simulink model "scale_model_model_control"  (R2024b)
settings: Solver=VariableStepAuto  StartTime=0.0  StopTime=100  MaxStep=0.02  RelTol=1e-3
values from neighbouring files (symbols this model uses):
  A_adrcl = [zeros(N, 1)  eye(N, N) ... (first row only)    [init_scale_blade_suspended_control.m]
  A_ESO_d = [1-l1_ESO_d, delta_t-l1_ESO_d*delta_t, 1/2 * delta_t^2 - 1/2 * l1_ESO_d*delta_t^2 ... (first row only)    [init_scale_blade_suspended_control.m]
  A_MESO_d = A_o_d - l_MESO_d*C_o_d*A_o_d    [init_scale_blade_suspended_control.m]
  b0 = 1.025    [init_scale_blade_suspended_control.m]
  b_adrcl = [zeros(N-1, 1) ... (first row only)    [init_scale_blade_suspended_control.m]
  b_ESO_d = [1/2*b0*delta_t^2 - l1_ESO_d*b0*delta_t^2 ... (first row only)    [init_scale_blade_suspended_control.m]
  B_MESO_d = B_o_d - l_MESO_d*C_o_d*B_o_d    [init_scale_blade_suspended_control.m]
  c_t = [1, zeros(1, N)]    [init_scale_blade_suspended_control.m]
  delta_t = 0.01    [init_scale_blade_suspended_control.m]
  DLADRC_max_effort = 30    [init_scale_blade_suspended_control.m]
  DLQRMADRC_max_effort = 30    [init_scale_blade_suspended_control.m]
  eta_s_init_n = [p_s_init_n;Theta_s_init_n]    [init_scale_blade_suspended_control.m]
  g = 9.81    [init_scale_blade_suspended_control.m]
  inv_M_s = inv(M_s)    [init_scale_blade_suspended_control.m]
  k = ones(N,1)    [init_scale_blade_suspended_control.m]
  k1_c_d = (1 - z_cl)^2/delta_t^2    [init_scale_blade_suspended_control.m]
  k_c_T_dlqr = dlqr(A_m_dlqr,b_m_dlqr,Q,R)    [init_scale_blade_suspended_control.m]
  k_d_T_lqr = (e_m*c_T_d_m_lqr) \ b_m_lqr    [init_scale_blade_suspended_control.m]
  k_s_lqr = -inv(c_T_m_lqr*inv(A_m_lqr-b_m_lqr*k_c_T_lqr)*b_m_lqr)    [init_scale_blade_suspended_control.m]
  k_T_d = [k1_c_d, k2_c_d]    [init_scale_blade_suspended_control.m]
  k_w1_s = gamma * EA/lw1_s_init    (= 19634.9540849)    [init_scale_blade_suspended_control.m]
  k_w2_s = k_w1_s    (= 19634.9540849)    [init_scale_blade_suspended_control.m]
  L = 0.8    [init_scale_blade_suspended_control.m]
  l = ones(N+1, 1)    [init_scale_blade_suspended_control.m]
  l_ESO_d = [l1_ESO_d, l2_ESO_d, l3_ESO_d]'    [init_scale_blade_suspended_control.m]
  l_MESO_d = acker(A_o_d',C_o_d',[z_MESO,z_MESO,z_MESO])'    [init_scale_blade_suspended_control.m]
  lw1_s_init = tot_liftWire-0.14    (= 0.56)    [init_scale_blade_suspended_control.m]
  lw2_s = norm(p_h_s_init- posSling_s_n(:,1))-elong_lw2_s    [init_scale_blade_suspended_control.m]
  m_h_s = 0.01    [init_scale_blade_suspended_control.m]
  meanWSP = 1    [init_scale_blade_suspended_control.m]
  N = 2    [init_scale_blade_suspended_control.m]
  nu_s_init_b = zeros(6,1)    [init_scale_blade_suspended_control.m]
  p_h_dot_s_init = [0;0;0]    [init_scale_blade_suspended_control.m]
  p_h_s_init = posCraneTip_s + [0;0;lw1_s_init + elong_mainlw_s]    [init_scale_blade_suspended_control.m]
  posCOG_s = [0;0;0]    [init_scale_blade_suspended_control.m]
  posCraneTip_s = [0;0;-1.2]    [init_scale_blade_suspended_control.m]
  posSling_s_b = [posCOG_s + [slings_p1_new(1); -0.05; slings_p1_new(2)],                posCOG_s + [slings_p1_new(1); 0.05; slings_p1_new(2)],               posCOG_s + [slings_p2_new(1); -0.05; slings_p2_new(2)],               posCOG_s + [slings_p2_new(1); 0.05; slings_p2_new(2)]]    [init_scale_blade_suspended_control.m]
  posThruster_s_b = [posCOG_s + [0.03; 0.21; -0.05],                posCOG_s + [0.03; -0.21; -0.05],               posCOG_s + [0; 0.1825; -0.05],               posCOG_s + [0; -0.1825; -0.05]]    [init_scale_blade_suspended_control.m]
  totalMass_s = 0.391    [init_scale_blade_suspended_control.m]
  W = 0.05    [init_scale_blade_suspended_control.m]
undefined symbols (not defined in the file or in its folder): A_o_dlqr, b_o_dlqr, c_o_T_dlqr, k_o_lqr, linsys_v2, sigbuilder_block
libraries: MarIn_blade x104, simulink_extras x28, slpidlib x5, simulink x4
(part 2 of 3)

== system scale_model_model_control/Discrete LADRC ==
  note: Discrete ESO
  ref : Inport
  y : Inport  Port=2
  Gain : Gain  Gain=l_ESO_d
  Gain1 : Gain  Gain=b_ESO_d
  Gain2 : Gain  Gain=A_ESO_d  Multiplication=Matrix(K*u)
  Gain3 : Gain  Gain=k1_c_d
  Gain4 : Gain  Gain=1/b0
  Gain5 : Gain  Gain=[k_T_d 1]  Multiplication=Matrix(K*u)
  Limiter : Saturate  UpperLimit=DLADRC_max_effort  LowerLimit=-DLADRC_max_effort
  Sum : Sum  Inputs=|+-
  Sum8 : Sum  Inputs=|++
  Sum9 : Sum  Inputs=+|+
  Unit Delay : UnitDelay  SampleTime=delta_t  HasFrameUpgradeWarning=on
  u : Outport
  wires:
  Gain1/1 -> Sum8/1
  Unit Delay/1 -> Sum9/1
  Sum8/1 -> Unit Delay/1
  Sum9/1 -> Gain5/1, Gain2/1  "x_hat"
  Gain/1 -> Sum9/2
  Gain2/1 -> Sum8/2
  Gain4/1 -> Limiter/1  "u"
  ref/1 -> Gain3/1
  Gain3/1 -> Sum/1
  Sum/1 -> Gain4/1
  Limiter/1 -> Gain1/1, u/1  "u_lim"
  y/1 -> Gain/1
  Gain5/1 -> Sum/2

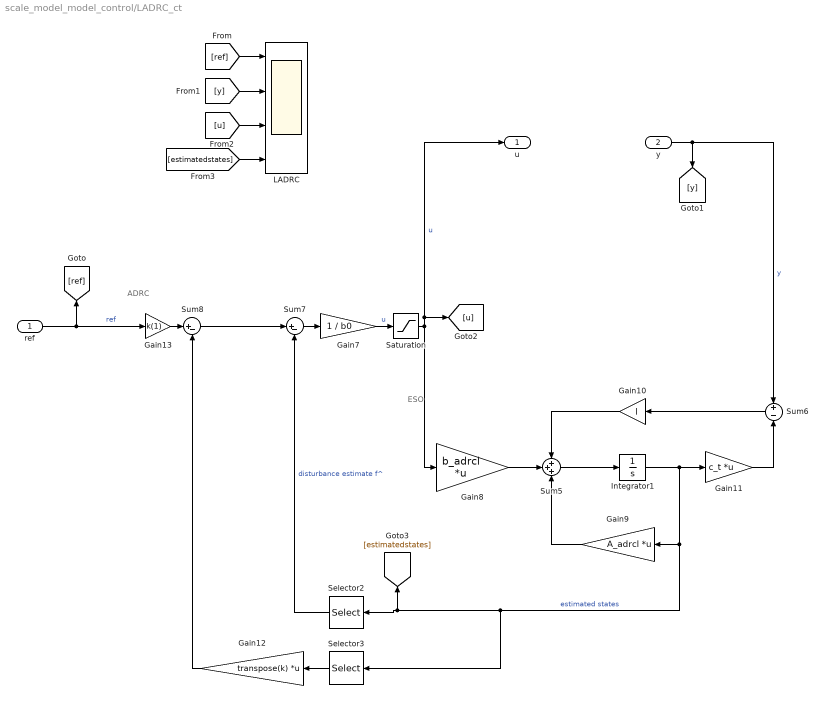
== system scale_model_model_control/LADRC_ct ==
  note: ESO
  note: ADRC
  ref : Inport
  y : Inport  Port=2
  Gain10 : Gain  Gain=l
  Gain11 : Gain  Gain=c_t  Multiplication=Matrix(K*u)
  Gain12 : Gain  Gain=transpose(k)  Multiplication=Matrix(K*u)
  Gain13 : Gain  Gain=k(1)
  Gain7 : Gain  Gain=1 / b0
  Gain8 : Gain  Gain=b_adrcl  Multiplication=Matrix(K*u)
  Gain9 : Gain  Gain=A_adrcl  Multiplication=Matrix(K*u)
  Integrator1 : Integrator
  LADRC : Scope  NumInputPorts=4
  Saturation : Saturate
  Selector2 : Selector  InputPortWidth=N+1  IndexOptions=Index vector (dialog)  Indices=[N+1]  OutputSizes=1
  Selector3 : Selector  InputPortWidth=N+1  IndexOptions=Index vector (dialog)  Indices=[1:N]  OutputSizes=1
  Sum5 : Sum  Inputs=+++
  Sum6 : Sum  Inputs=+|-
  Sum7 : Sum  Inputs=|+-
  Sum8 : Sum  Inputs=|+-
  u : Outport
  wires:
  Gain8/1 -> Sum5/2
  Saturation/1 -> u/1, [u], Gain8/1  "u"
  Integrator1/1 -> Gain11/1, Selector3/1, [estimatedstates], Selector2/1, Gain9/1  "estimated states"
  Gain11/1 -> Sum6/2
  Sum6/1 -> Gain10/1
  Selector2/1 -> Sum7/2  "disturbance estimate f^"
  Sum7/1 -> Gain7/1
  Gain12/1 -> Sum8/2
  Gain10/1 -> Sum5/1
  Gain9/1 -> Sum5/3
  Gain13/1 -> Sum8/1
  Sum5/1 -> Integrator1/1
  Selector3/1 -> Gain12/1
  Sum8/1 -> Sum7/1
  ref/1 -> [ref], Gain13/1  "ref"
  y/1 -> Sum6/1, [y]  "y"
  [ref] -> LADRC/1
  [y] -> LADRC/2
  [u] -> LADRC/3
  [estimatedstates] -> LADRC/4
  Gain7/1 -> Saturation/1  "u"

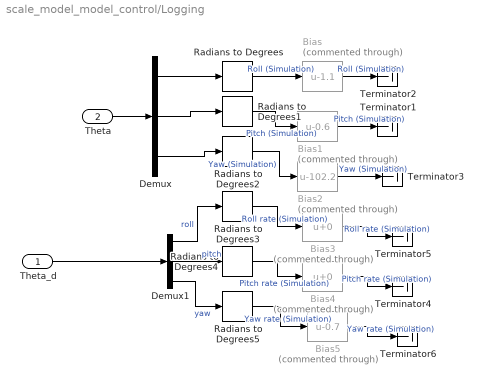
== system scale_model_model_control/Logging ==
  Theta_d : Inport
  Theta : Inport  Port=2
  Bias : Bias  Commented=through  Bias=-1.1  SaturateOnIntegerOverflow=off
  Bias1 : Bias  Commented=through  Bias=-0.6  SaturateOnIntegerOverflow=off
  Bias2 : Bias  Commented=through  Bias=-102.2  SaturateOnIntegerOverflow=off
  Bias3 : Bias  Commented=through  SaturateOnIntegerOverflow=off
  Bias4 : Bias  Commented=through  SaturateOnIntegerOverflow=off
  Bias5 : Bias  Commented=through  Bias=-0.7  SaturateOnIntegerOverflow=off
  Demux : Demux  Outputs=3
  Demux1 : Demux  Outputs=3
  Radians to Degrees{,1..5} (6 alike) : simulink_extras/Transformations/Radians to Degrees
  Terminator{1..6} (6 alike) : Terminator
  wires:
  Bias5/1 -> Terminator6/1  "Yaw rate (Simulation)"
  Bias2/1 -> Terminator3/1  "Yaw (Simulation)"
  Radians to Degrees3/1 -> Bias3/1  "Roll rate (Simulation)"
  Radians to Degrees5/1 -> Bias5/1  "Yaw rate (Simulation)"
  Bias/1 -> Terminator2/1  "Roll (Simulation)"
  Radians to Degrees/1 -> Bias/1  "Roll (Simulation)"
  Bias3/1 -> Terminator5/1  "Roll rate (Simulation)"
  Radians to Degrees4/1 -> Bias4/1  "Pitch rate (Simulation)"
  Demux1/3 -> Radians to Degrees5/1  "yaw"
  Demux1/1 -> Radians to Degrees3/1  "roll"
  Radians to Degrees2/1 -> Bias2/1  "Yaw (Simulation)"
  Bias4/1 -> Terminator4/1  "Pitch rate (Simulation)"
  Bias1/1 -> Terminator1/1  "Pitch (Simulation)"
  Radians to Degrees1/1 -> Bias1/1  "Pitch (Simulation)"
  Demux1/2 -> Radians to Degrees4/1  "pitch"
  Theta_d/1 -> Demux1/1
  Theta/1 -> Demux/1
  Demux/1 -> Radians to Degrees/1
  Demux/2 -> Radians to Degrees1/1
  Demux/3 -> Radians to Degrees2/1

== system scale_model_model_control/Logging1 ==
  Theta_d : Inport
  Theta : Inport  Port=2
  Bias : Bias  Commented=through  Bias=-1.1  SaturateOnIntegerOverflow=off
  Bias1 : Bias  Commented=through  Bias=-0.6  SaturateOnIntegerOverflow=off
  Bias2 : Bias  Commented=through  Bias=-102.2  SaturateOnIntegerOverflow=off
  Bias3 : Bias  Commented=through  SaturateOnIntegerOverflow=off
  Bias4 : Bias  Commented=through  SaturateOnIntegerOverflow=off
  Bias5 : Bias  Commented=through  Bias=-0.7  SaturateOnIntegerOverflow=off
  Demux : Demux  Outputs=3
  Demux1 : Demux  Outputs=3
  Radians to Degrees{,1..5} (6 alike) : simulink_extras/Transformations/Radians to Degrees
  Terminator{1..6} (6 alike) : Terminator
  wires:
  Bias5/1 -> Terminator6/1  "Yaw rate (Simulation)"
  Bias2/1 -> Terminator3/1  "Yaw (Simulation)"
  Radians to Degrees3/1 -> Bias3/1  "Roll rate (Simulation)"
  Radians to Degrees5/1 -> Bias5/1  "Yaw rate (Simulation)"
  Bias/1 -> Terminator2/1  "Roll (Simulation)"
  Radians to Degrees/1 -> Bias/1  "Roll (Simulation)"
  Bias3/1 -> Terminator5/1  "Roll rate (Simulation)"
  Radians to Degrees4/1 -> Bias4/1  "Pitch rate (Simulation)"
  Demux1/3 -> Radians to Degrees5/1  "yaw"
  Demux1/1 -> Radians to Degrees3/1  "roll"
  Radians to Degrees2/1 -> Bias2/1  "Yaw (Simulation)"
  Bias4/1 -> Terminator4/1  "Pitch rate (Simulation)"
  Bias1/1 -> Terminator1/1  "Pitch (Simulation)"
  Radians to Degrees1/1 -> Bias1/1  "Pitch (Simulation)"
  Demux1/2 -> Radians to Degrees4/1  "pitch"
  Theta_d/1 -> Demux1/1
  Theta/1 -> Demux/1
  Demux/1 -> Radians to Degrees/1
  Demux/2 -> Radians to Degrees1/1
  Demux/3 -> Radians to Degrees2/1

== system scale_model_model_control/Logging2 ==
  Theta_d : Inport
  Theta : Inport  Port=2
  Bias : Bias  Commented=through  Bias=-1.1  SaturateOnIntegerOverflow=off
  Bias1 : Bias  Commented=through  Bias=-0.6  SaturateOnIntegerOverflow=off
  Bias2 : Bias  Commented=through  Bias=-102.2  SaturateOnIntegerOverflow=off
  Bias3 : Bias  Commented=through  SaturateOnIntegerOverflow=off
  Bias4 : Bias  Commented=through  SaturateOnIntegerOverflow=off
  Bias5 : Bias  Commented=through  Bias=-0.7  SaturateOnIntegerOverflow=off
  Demux : Demux  Outputs=3
  Demux1 : Demux  Outputs=3
  Radians to Degrees{,1..5} (6 alike) : simulink_extras/Transformations/Radians to Degrees
  Terminator{1..6} (6 alike) : Terminator
  wires:
  Bias5/1 -> Terminator6/1  "Yaw rate (Simulation)"
  Bias2/1 -> Terminator3/1  "Yaw (Simulation)"
  Radians to Degrees3/1 -> Bias3/1  "Roll rate (Simulation)"
  Radians to Degrees5/1 -> Bias5/1  "Yaw rate (Simulation)"
  Bias/1 -> Terminator2/1  "Roll (Simulation)"
  Radians to Degrees/1 -> Bias/1  "Roll (Simulation)"
  Bias3/1 -> Terminator5/1  "Roll rate (Simulation)"
  Radians to Degrees4/1 -> Bias4/1  "Pitch rate (Simulation)"
  Demux1/3 -> Radians to Degrees5/1  "yaw"
  Demux1/1 -> Radians to Degrees3/1  "roll"
  Radians to Degrees2/1 -> Bias2/1  "Yaw (Simulation)"
  Bias4/1 -> Terminator4/1  "Pitch rate (Simulation)"
  Bias1/1 -> Terminator1/1  "Pitch (Simulation)"
  Radians to Degrees1/1 -> Bias1/1  "Pitch (Simulation)"
  Demux1/2 -> Radians to Degrees4/1  "pitch"
  Theta_d/1 -> Demux1/1
  Theta/1 -> Demux/1
  Demux/1 -> Radians to Degrees/1
  Demux/2 -> Radians to Degrees1/1
  Demux/3 -> Radians to Degrees2/1

== system scale_model_model_control/Logging3 ==
  Theta_d : Inport
  Theta : Inport  Port=2
  Bias : Bias  Commented=through  Bias=-1.1  SaturateOnIntegerOverflow=off
  Bias1 : Bias  Commented=through  Bias=-0.6  SaturateOnIntegerOverflow=off
  Bias2 : Bias  Commented=through  Bias=-102.2  SaturateOnIntegerOverflow=off
  Bias3 : Bias  Commented=through  SaturateOnIntegerOverflow=off
  Bias4 : Bias  Commented=through  SaturateOnIntegerOverflow=off
  Bias5 : Bias  Commented=through  Bias=-0.7  SaturateOnIntegerOverflow=off
  Demux : Demux  Outputs=3
  Demux1 : Demux  Outputs=3
  Radians to Degrees{,1..5} (6 alike) : simulink_extras/Transformations/Radians to Degrees
  Terminator{1..6} (6 alike) : Terminator
  wires:
  Bias5/1 -> Terminator6/1  "Yaw rate (Simulation)"
  Bias2/1 -> Terminator3/1  "Yaw (Simulation)"
  Radians to Degrees3/1 -> Bias3/1  "Roll rate (Simulation)"
  Radians to Degrees5/1 -> Bias5/1  "Yaw rate (Simulation)"
  Bias/1 -> Terminator2/1  "Roll (Simulation)"
  Radians to Degrees/1 -> Bias/1  "Roll (Simulation)"
  Bias3/1 -> Terminator5/1  "Roll rate (Simulation)"
  Radians to Degrees4/1 -> Bias4/1  "Pitch rate (Simulation)"
  Demux1/3 -> Radians to Degrees5/1  "yaw"
  Demux1/1 -> Radians to Degrees3/1  "roll"
  Radians to Degrees2/1 -> Bias2/1  "Yaw (Simulation)"
  Bias4/1 -> Terminator4/1  "Pitch rate (Simulation)"
  Bias1/1 -> Terminator1/1  "Pitch (Simulation)"
  Radians to Degrees1/1 -> Bias1/1  "Pitch (Simulation)"
  Demux1/2 -> Radians to Degrees4/1  "pitch"
  Theta_d/1 -> Demux1/1
  Theta/1 -> Demux/1
  Demux/1 -> Radians to Degrees/1
  Demux/2 -> Radians to Degrees1/1
  Demux/3 -> Radians to Degrees2/1

== system scale_model_model_control/Thrusters ==
  M_Tx : Inport
  M_Tz : Inport  Port=2
  Abs : Abs  SaturateOnIntegerOverflow=off
  Abs1 : Abs  SaturateOnIntegerOverflow=off
  Constant : Constant  Value=0
  Constant1 : Constant  Value=posThruster_s_b(2,2)
  Divide : Product  Inputs=*/
  Divide1 : Product  Inputs=*/
  Max F_t ~0.3N : Saturate  UpperLimit=0.076  LowerLimit=-0.076  LinearizeAsGain=off
  Mux : Mux
  Mux{1..4} (4 alike) : Mux  Inputs=3
  Saturation : Saturate  UpperLimit=0  LowerLimit=-inf
  Saturation1 : Saturate  UpperLimit=inf  LowerLimit=0
  Saturation2 : Saturate  UpperLimit=0  LowerLimit=-inf
  Saturation3 : Saturate  UpperLimit=inf  LowerLimit=0
  "F_thrusters {b}" : Outport
  wires:
  Mux1/1 -> Mux/1  "thruster1 (yaw)"
  Mux2/1 -> Mux/2  "thruster2 (yaw)"
  Mux3/1 -> Mux/3  "thruster3 (roll)"
  Mux4/1 -> Mux/4  "thruster4 (roll)"
  Constant/1 -> Mux1/3, Mux3/1, Mux4/2, Mux4/1, Mux3/2, Mux2/3, Mux2/2, Mux1/2
  M_Tx/1 -> Divide/1
  Constant1/1 -> Divide1/2, Divide/2
  M_Tz/1 -> Divide1/1
  Divide1/1 -> Saturation/1, Saturation1/1
  Saturation1/1 -> Mux1/1
  Saturation/1 -> Abs1/1
  Divide/1 -> Saturation2/1, Saturation3/1
  Saturation3/1 -> Mux4/3
  Saturation2/1 -> Abs/1
  Abs/1 -> Mux3/3
  Abs1/1 -> Mux2/1
  Mux/1 -> Max F_t ~0.3N/1
  Max F_t ~0.3N/1 -> "F_thrusters {b}"/1  "F_T"

== system scale_model_model_control/Thrusters1 ==
  M_Tx : Inport
  M_Tz : Inport  Port=2
  Abs : Abs  SaturateOnIntegerOverflow=off
  Abs1 : Abs  SaturateOnIntegerOverflow=off
  Constant : Constant  Value=0
  Constant1 : Constant  Value=posThruster_s_b(2,2)
  Divide : Product  Inputs=*/
  Divide1 : Product  Inputs=*/
  Max F_t ~0.3N : Saturate  UpperLimit=0.076  LowerLimit=-0.076  LinearizeAsGain=off
  Mux : Mux
  Mux{1..4} (4 alike) : Mux  Inputs=3
  Saturation : Saturate  UpperLimit=0  LowerLimit=-inf
  Saturation1 : Saturate  UpperLimit=inf  LowerLimit=0
  Saturation2 : Saturate  UpperLimit=0  LowerLimit=-inf
  Saturation3 : Saturate  UpperLimit=inf  LowerLimit=0
  "F_thrusters {b}" : Outport
  wires:
  Mux1/1 -> Mux/1  "thruster1 (yaw)"
  Mux2/1 -> Mux/2  "thruster2 (yaw)"
  Mux3/1 -> Mux/3  "thruster3 (roll)"
  Mux4/1 -> Mux/4  "thruster4 (roll)"
  Constant/1 -> Mux1/3, Mux3/1, Mux4/2, Mux4/1, Mux3/2, Mux2/3, Mux2/2, Mux1/2
  M_Tx/1 -> Divide/1
  Constant1/1 -> Divide1/2, Divide/2
  M_Tz/1 -> Divide1/1
  Divide1/1 -> Saturation/1, Saturation1/1
  Saturation1/1 -> Mux1/1
  Saturation/1 -> Abs1/1
  Divide/1 -> Saturation2/1, Saturation3/1
  Saturation3/1 -> Mux4/3
  Saturation2/1 -> Abs/1
  Abs/1 -> Mux3/3
  Abs1/1 -> Mux2/1
  Mux/1 -> Max F_t ~0.3N/1
  Max F_t ~0.3N/1 -> "F_thrusters {b}"/1  "F_T"

== system scale_model_model_control/Thrusters2 ==
  M_Tx : Inport
  M_Tz : Inport  Port=2
  Abs : Abs  SaturateOnIntegerOverflow=off
  Abs1 : Abs  SaturateOnIntegerOverflow=off
  Constant : Constant  Value=0
  Constant1 : Constant  Value=posThruster_s_b(2,2)
  Divide : Product  Inputs=*/
  Divide1 : Product  Inputs=*/
  Max F_t ~0.3N : Saturate  UpperLimit=0.076  LowerLimit=-0.076  LinearizeAsGain=off
  Mux : Mux
  Mux{1..4} (4 alike) : Mux  Inputs=3
  Saturation : Saturate  UpperLimit=0  LowerLimit=-inf
  Saturation1 : Saturate  UpperLimit=inf  LowerLimit=0
  Saturation2 : Saturate  UpperLimit=0  LowerLimit=-inf
  Saturation3 : Saturate  UpperLimit=inf  LowerLimit=0
  "F_thrusters {b}" : Outport
  wires:
  Mux1/1 -> Mux/1  "thruster1 (yaw)"
  Mux2/1 -> Mux/2  "thruster2 (yaw)"
  Mux3/1 -> Mux/3  "thruster3 (roll)"
  Mux4/1 -> Mux/4  "thruster4 (roll)"
  Constant/1 -> Mux1/3, Mux3/1, Mux4/2, Mux4/1, Mux3/2, Mux2/3, Mux2/2, Mux1/2
  M_Tx/1 -> Divide/1
  Constant1/1 -> Divide1/2, Divide/2
  M_Tz/1 -> Divide1/1
  Divide1/1 -> Saturation/1, Saturation1/1
  Saturation1/1 -> Mux1/1
  Saturation/1 -> Abs1/1
  Divide/1 -> Saturation2/1, Saturation3/1
  Saturation3/1 -> Mux4/3
  Saturation2/1 -> Abs/1
  Abs/1 -> Mux3/3
  Abs1/1 -> Mux2/1
  Mux/1 -> Max F_t ~0.3N/1
  Max F_t ~0.3N/1 -> "F_thrusters {b}"/1  "F_T"

== system scale_model_model_control/Thrusters3 ==
  M_Tx : Inport
  M_Tz : Inport  Port=2
  Abs : Abs  SaturateOnIntegerOverflow=off
  Abs1 : Abs  SaturateOnIntegerOverflow=off
  Constant : Constant  Value=0
  Constant1 : Constant  Value=posThruster_s_b(2,2)
  Divide : Product  Inputs=*/
  Divide1 : Product  Inputs=*/
  Max F_t ~0.3N : Saturate  UpperLimit=0.076  LowerLimit=-0.076  LinearizeAsGain=off
  Mux : Mux
  Mux{1..4} (4 alike) : Mux  Inputs=3
  Saturation : Saturate  UpperLimit=0  LowerLimit=-inf
  Saturation1 : Saturate  UpperLimit=inf  LowerLimit=0
  Saturation2 : Saturate  UpperLimit=0  LowerLimit=-inf
  Saturation3 : Saturate  UpperLimit=inf  LowerLimit=0
  "F_thrusters {b}" : Outport
  wires:
  Mux1/1 -> Mux/1  "thruster1 (yaw)"
  Mux2/1 -> Mux/2  "thruster2 (yaw)"
  Mux3/1 -> Mux/3  "thruster3 (roll)"
  Mux4/1 -> Mux/4  "thruster4 (roll)"
  Constant/1 -> Mux1/3, Mux3/1, Mux4/2, Mux4/1, Mux3/2, Mux2/3, Mux2/2, Mux1/2
  M_Tx/1 -> Divide/1
  Constant1/1 -> Divide1/2, Divide/2
  M_Tz/1 -> Divide1/1
  Divide1/1 -> Saturation/1, Saturation1/1
  Saturation1/1 -> Mux1/1
  Saturation/1 -> Abs1/1
  Divide/1 -> Saturation2/1, Saturation3/1
  Saturation3/1 -> Mux4/3
  Saturation2/1 -> Abs/1
  Abs/1 -> Mux3/3
  Abs1/1 -> Mux2/1
  Mux/1 -> Max F_t ~0.3N/1
  Max F_t ~0.3N/1 -> "F_thrusters {b}"/1  "F_T"

== system scale_model_model_control/Blade+Yoke/Signal Builder2 ==
  Demux : Demux  Tag=STV Demux  Outputs=1
      settings: DisplayOption=none
  FromWs : FromWorkspace  Tag=STV FromWs  VariableName=tuvar
      SigBuilderData=|
      | common.afterFinalStr = 'Extrapolate'
      | common.sampleTime = 0
      | dataSet.timeRange = [0 10]
      | dataSet.name = 'Group 1'
      | sbobj.Groups.Name = 'Group 1'
      | sbobj.Groups.Signals.Name = 'Signal 1'
      | sbobj.Groups.Signals.XData = [0 2 2 2.1 2.1 10]
      | sbobj.Groups.Signals.YData = [0 0 1 1 0 0]
  Signal 1 : Outport  Tag=STV Outport
  wires:
  Demux/1 -> Signal 1/1
  FromWs/1 -> Demux/1

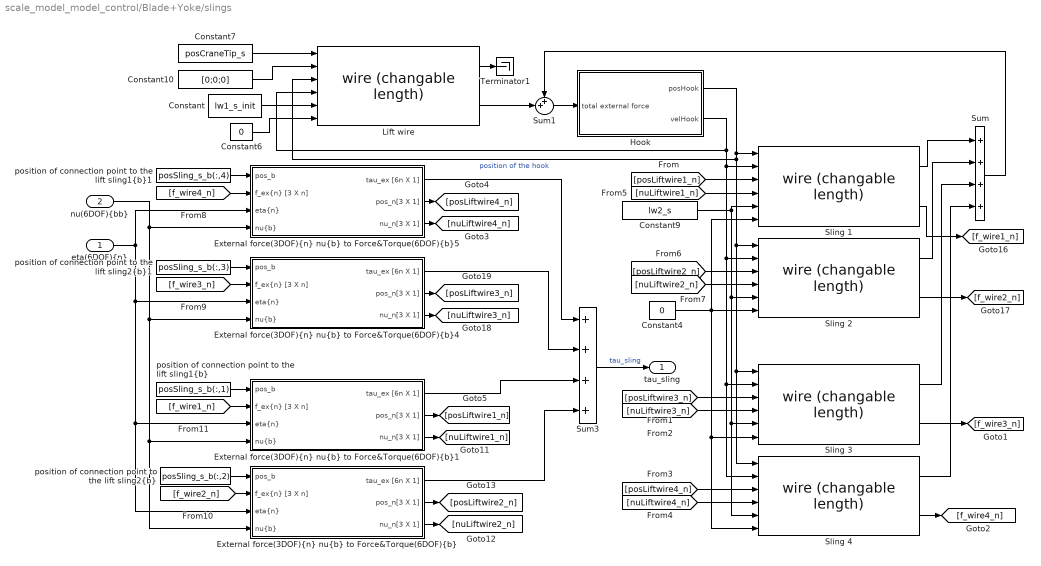
== system scale_model_model_control/Blade+Yoke/slings ==
  "eta(6DOF){n}" : Inport
  "nu(6DOF){bb}" : Inport  Port=2
  Constant : Constant  Value=lw1_s_init
  Constant10 : Constant  Value=[0;0;0]
  Constant4 : Constant  Value=0
  Constant6 : Constant  Value=0
  Constant7 : Constant  Value=posCraneTip_s
  Constant9 : Constant  Value=lw2_s
  "External force(3DOF){n} nu{b} to Force&Torque(6DOF){b}" : Subsystem  AncestorBlock=MarIn_blade/Basic functions/External force(3DOF){n} nu{b} to Force&Torque(6DOF){b}  mask(External force(3DOF){n} nu{b} to Force&Torque(6DOF){b}){}
      mask help:
      | Translate position and velocity in {b} to {n}.
      |
      |
      | Author: Zhengru Ren
      | Date: April 22, 2017
  "External force(3DOF){n} nu{b} to Force&Torque(6DOF){b}1" : Subsystem  AncestorBlock=MarIn_blade/Basic functions/External force(3DOF){n} nu{b} to Force&Torque(6DOF){b}  mask(External force(3DOF){n} nu{b} to Force&Torque(6DOF){b}){}
      mask help:
      | Translate position and velocity in {b} to {n}.
      |
      |
      | Author: Zhengru Ren
      | Date: April 22, 2017
  "External force(3DOF){n} nu{b} to Force&Torque(6DOF){b}4" : Subsystem  AncestorBlock=MarIn_blade/Basic functions/External force(3DOF){n} nu{b} to Force&Torque(6DOF){b}  mask(External force(3DOF){n} nu{b} to Force&Torque(6DOF){b}){}
      mask help:
      | Translate position and velocity in {b} to {n}.
      |
      |
      | Author: Zhengru Ren
      | Date: April 22, 2017
  "External force(3DOF){n} nu{b} to Force&Torque(6DOF){b}5" : Subsystem  AncestorBlock=MarIn_blade/Basic functions/External force(3DOF){n} nu{b} to Force&Torque(6DOF){b}  mask(External force(3DOF){n} nu{b} to Force&Torque(6DOF){b}){}
      mask help:
      | Translate position and velocity in {b} to {n}.
      |
      |
      | Author: Zhengru Ren
      | Date: April 22, 2017
  Hook : Subsystem  AncestorBlock=|  mask(Hook){m_h=m_h_s, p_h_init=p_h_s_init, p_h_dot_init=p_h_dot_s_init}
      | MarIn_blade/Lifting equipments
      | (winch, wire, hook)/Hook
      mask prompts: m_h "Hook mass (m_h) [kg]"; p_h_init "Initial position of the hook"; p_h_dot_init "Initial velocity of the hook"
      mask help:
      | Used to simulate a hook.
      |
      | Author: Zhengru Ren
      | Date: May 20, 2016
      mask init:
      | invM_h = diag([1/m_h,1/m_h,1/m_h]);
  Lift wire : MarIn_blade/Lifting equipments (winch, wire, hook)/wire (changable length)  k=k_w1_s  c=d_w1_s
      settings: SourceProductName=MarIn (Blade)
  Sling {1..4} (4 alike) : MarIn_blade/Lifting equipments (winch, wire, hook)/wire (changable length)  k=k_w2_s  c=d_w2_s
      settings: SourceProductName=MarIn (Blade)
  Sum : Sum  Inputs=++++
  Sum1 : Sum  Inputs=++|
  Sum3 : Sum  Inputs=4
  Terminator1 : Terminator
  "position of connection point to the lift sling1{b}" : Constant  Value=posSling_s_b(:,1)
  "position of connection point to the lift sling1{b}1" : Constant  Value=posSling_s_b(:,4)
  "position of connection point to the lift sling2{b}" : Constant  Value=posSling_s_b(:,2)
  "position of connection point to the lift sling2{b}1" : Constant  Value=posSling_s_b(:,3)
  tau_sling : Outport
  wires:
  "nu(6DOF){bb}"/1 -> "External force(3DOF){n} nu{b} to Force&Torque(6DOF){b}"/4("nu{b}"), "External force(3DOF){n} nu{b} to Force&Torque(6DOF){b}1"/4("nu{b}"), "External force(3DOF){n} nu{b} to Force&Torque(6DOF){b}4"/4("nu{b}"), "External force(3DOF){n} nu{b} to Force&Torque(6DOF){b}5"/4("nu{b}")
  "position of connection point to the lift sling1{b}1"/1 -> "External force(3DOF){n} nu{b} to Force&Torque(6DOF){b}5"/1(pos_b)
  "External force(3DOF){n} nu{b} to Force&Torque(6DOF){b}"/1(tau_ex [6n X 1]) -> Sum3/4
  "eta(6DOF){n}"/1 -> "External force(3DOF){n} nu{b} to Force&Torque(6DOF){b}5"/3("eta{n}"), "External force(3DOF){n} nu{b} to Force&Torque(6DOF){b}"/3("eta{n}"), "External force(3DOF){n} nu{b} to Force&Torque(6DOF){b}1"/3("eta{n}"), "External force(3DOF){n} nu{b} to Force&Torque(6DOF){b}4"/3("eta{n}")
  "External force(3DOF){n} nu{b} to Force&Torque(6DOF){b}5"/1(tau_ex [6n X 1]) -> Sum3/1
  "position of connection point to the lift sling2{b}"/1 -> "External force(3DOF){n} nu{b} to Force&Torque(6DOF){b}"/1(pos_b)
  Sum3/1 -> tau_sling/1  "tau_sling"
  "External force(3DOF){n} nu{b} to Force&Torque(6DOF){b}4"/1(tau_ex [6n X 1]) -> Sum3/2
  [f_wire4_n] -> "External force(3DOF){n} nu{b} to Force&Torque(6DOF){b}5"/2("f_ex{n} [3 X n]")
  [f_wire3_n] -> "External force(3DOF){n} nu{b} to Force&Torque(6DOF){b}4"/2("f_ex{n} [3 X n]")
  "position of connection point to the lift sling2{b}1"/1 -> "External force(3DOF){n} nu{b} to Force&Torque(6DOF){b}4"/1(pos_b)
  "External force(3DOF){n} nu{b} to Force&Torque(6DOF){b}1"/3(nu_n[3 X 1]) -> [nuLiftwire1_n]
  "External force(3DOF){n} nu{b} to Force&Torque(6DOF){b}4"/2(pos_n[3 X 1]) -> [posLiftwire3_n]
  "position of connection point to the lift sling1{b}"/1 -> "External force(3DOF){n} nu{b} to Force&Torque(6DOF){b}1"/1(pos_b)
  "External force(3DOF){n} nu{b} to Force&Torque(6DOF){b}4"/3(nu_n[3 X 1]) -> [nuLiftwire3_n]
  [f_wire2_n] -> "External force(3DOF){n} nu{b} to Force&Torque(6DOF){b}"/2("f_ex{n} [3 X n]")
  "External force(3DOF){n} nu{b} to Force&Torque(6DOF){b}"/3(nu_n[3 X 1]) -> [nuLiftwire2_n]
  "External force(3DOF){n} nu{b} to Force&Torque(6DOF){b}"/2(pos_n[3 X 1]) -> [posLiftwire2_n]
  "External force(3DOF){n} nu{b} to Force&Torque(6DOF){b}1"/1(tau_ex [6n X 1]) -> Sum3/3
  "External force(3DOF){n} nu{b} to Force&Torque(6DOF){b}1"/2(pos_n[3 X 1]) -> [posLiftwire1_n]
  [f_wire1_n] -> "External force(3DOF){n} nu{b} to Force&Torque(6DOF){b}1"/2("f_ex{n} [3 X n]")
  Sling 4/2 -> [f_wire4_n]
  Sling 3/2 -> [f_wire3_n]
  Sling 4/1 -> Sum/4
  Sling 3/1 -> Sum/3
  [posLiftwire3_n] -> Sling 3/3
  [nuLiftwire3_n] -> Sling 3/4
  Hook/2(velHook) -> Sling 3/2, Sling 4/2, Sling 2/2, Sling 1/2, Lift wire/4
  Constant/1 -> Lift wire/5
  [posLiftwire1_n] -> Sling 1/3
  Sling 1/2 -> [f_wire1_n]
  [nuLiftwire1_n] -> Sling 1/4
  Sling 2/1 -> Sum/2
  Sling 2/2 -> [f_wire2_n]
  [posLiftwire2_n] -> Sling 2/3
  [nuLiftwire2_n] -> Sling 2/4
  Constant9/1 -> Sling 1/5, Sling 2/5, Sling 3/5, Sling 4/5
  Constant7/1 -> Lift wire/1
  Constant10/1 -> Lift wire/2
  Sum/1 -> Sum1/1
  Lift wire/2 -> Sum1/2
  Lift wire/1 -> Terminator1/1
  Sum1/1 -> Hook/1(total external force)
  Hook/1(posHook) -> Sling 3/1, Sling 4/1, Sling 2/1, Lift wire/3, Sling 1/1  "position of the hook"
  Constant4/1 -> Sling 2/6, Sling 1/6, Sling 3/6, Sling 4/6
  Constant6/1 -> Lift wire/6
  Sling 1/1 -> Sum/1
  [nuLiftwire4_n] -> Sling 4/4
  [posLiftwire4_n] -> Sling 4/3
  "External force(3DOF){n} nu{b} to Force&Torque(6DOF){b}5"/3(nu_n[3 X 1]) -> [nuLiftwire4_n]
  "External force(3DOF){n} nu{b} to Force&Torque(6DOF){b}5"/2(pos_n[3 X 1]) -> [posLiftwire4_n]

== system scale_model_model_control/Blade+Yoke/thrusters ==
  "F_thrusters {b}" : Inport
  Demux : Demux
  Force(3DOF){b}2Force&Torque(6DOF){b}{,1..3} (4 alike) : MarIn_blade/Basic functions/Force(3DOF){b}2Force&Torque(6DOF){b}  posCOG_bb=posCOG_s
      settings: SourceProductName=MarIn (Blade)
  Sum3 : Sum  Inputs=4
  "position of connection point to thruster1{b}" : Constant  Value=posThruster_s_b(:,1)
  "position of connection point to thruster2{b}" : Constant  Value=posThruster_s_b(:,2)
  "position of connection point to thruster3{b}" : Constant  Value=posThruster_s_b(:,3)
  "position of connection point to thruster4{b}" : Constant  Value=posThruster_s_b(:,4)
  tau_thrusters : Outport
  wires:
  "position of connection point to thruster1{b}"/1 -> "Force(3DOF){b}2Force&Torque(6DOF){b}1"/1
  "position of connection point to thruster3{b}"/1 -> "Force(3DOF){b}2Force&Torque(6DOF){b}2"/1
  Sum3/1 -> tau_thrusters/1  "tau_thrusters"
  "position of connection point to thruster2{b}"/1 -> "Force(3DOF){b}2Force&Torque(6DOF){b}"/1
  "Force(3DOF){b}2Force&Torque(6DOF){b}"/1 -> Sum3/4
  "position of connection point to thruster4{b}"/1 -> "Force(3DOF){b}2Force&Torque(6DOF){b}3"/1
  "Force(3DOF){b}2Force&Torque(6DOF){b}3"/1 -> Sum3/1
  "Force(3DOF){b}2Force&Torque(6DOF){b}2"/1 -> Sum3/2
  "Force(3DOF){b}2Force&Torque(6DOF){b}1"/1 -> Sum3/3
  "F_thrusters {b}"/1 -> Demux/1
  Demux/4 -> "Force(3DOF){b}2Force&Torque(6DOF){b}3"/2
  Demux/3 -> "Force(3DOF){b}2Force&Torque(6DOF){b}2"/2
  Demux/1 -> "Force(3DOF){b}2Force&Torque(6DOF){b}1"/2
  Demux/2 -> "Force(3DOF){b}2Force&Torque(6DOF){b}"/2

== system scale_model_model_control/Blade+Yoke1/Signal Builder2 ==
  Demux : Demux  Tag=STV Demux  Outputs=1
      settings: DisplayOption=none
  FromWs : FromWorkspace  Tag=STV FromWs  VariableName=tuvar
      SigBuilderData=|
      | common.afterFinalStr = 'Extrapolate'
      | common.sampleTime = 0
      | dataSet.timeRange = [0 10]
      | dataSet.name = 'Group 1'
      | sbobj.Groups.Name = 'Group 1'
      | sbobj.Groups.Signals.Name = 'Signal 1'
      | sbobj.Groups.Signals.XData = [0 2 2 2.1 2.1 10]
      | sbobj.Groups.Signals.YData = [0 0 1 1 0 0]
  Signal 1 : Outport  Tag=STV Outport
  wires:
  Demux/1 -> Signal 1/1
  FromWs/1 -> Demux/1

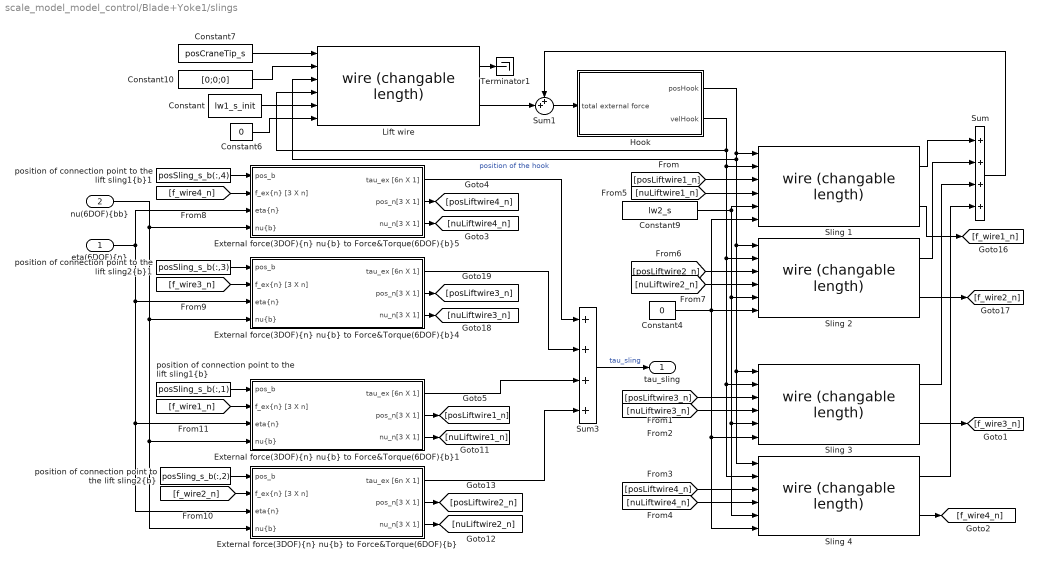
== system scale_model_model_control/Blade+Yoke1/slings ==
  "eta(6DOF){n}" : Inport
  "nu(6DOF){bb}" : Inport  Port=2
  Constant : Constant  Value=lw1_s_init
  Constant10 : Constant  Value=[0;0;0]
  Constant4 : Constant  Value=0
  Constant6 : Constant  Value=0
  Constant7 : Constant  Value=posCraneTip_s
  Constant9 : Constant  Value=lw2_s
  "External force(3DOF){n} nu{b} to Force&Torque(6DOF){b}" : Subsystem  AncestorBlock=MarIn_blade/Basic functions/External force(3DOF){n} nu{b} to Force&Torque(6DOF){b}  mask(External force(3DOF){n} nu{b} to Force&Torque(6DOF){b}){}
      mask help:
      | Translate position and velocity in {b} to {n}.
      |
      |
      | Author: Zhengru Ren
      | Date: April 22, 2017
  "External force(3DOF){n} nu{b} to Force&Torque(6DOF){b}1" : Subsystem  AncestorBlock=MarIn_blade/Basic functions/External force(3DOF){n} nu{b} to Force&Torque(6DOF){b}  mask(External force(3DOF){n} nu{b} to Force&Torque(6DOF){b}){}
      mask help:
      | Translate position and velocity in {b} to {n}.
      |
      |
      | Author: Zhengru Ren
      | Date: April 22, 2017
  "External force(3DOF){n} nu{b} to Force&Torque(6DOF){b}4" : Subsystem  AncestorBlock=MarIn_blade/Basic functions/External force(3DOF){n} nu{b} to Force&Torque(6DOF){b}  mask(External force(3DOF){n} nu{b} to Force&Torque(6DOF){b}){}
      mask help:
      | Translate position and velocity in {b} to {n}.
      |
      |
      | Author: Zhengru Ren
      | Date: April 22, 2017
  "External force(3DOF){n} nu{b} to Force&Torque(6DOF){b}5" : Subsystem  AncestorBlock=MarIn_blade/Basic functions/External force(3DOF){n} nu{b} to Force&Torque(6DOF){b}  mask(External force(3DOF){n} nu{b} to Force&Torque(6DOF){b}){}
      mask help:
      | Translate position and velocity in {b} to {n}.
      |
      |
      | Author: Zhengru Ren
      | Date: April 22, 2017
  Hook : Subsystem  AncestorBlock=|  mask(Hook){m_h=m_h_s, p_h_init=p_h_s_init, p_h_dot_init=p_h_dot_s_init}
      | MarIn_blade/Lifting equipments
      | (winch, wire, hook)/Hook
      mask prompts: m_h "Hook mass (m_h) [kg]"; p_h_init "Initial position of the hook"; p_h_dot_init "Initial velocity of the hook"
      mask help:
      | Used to simulate a hook.
      |
      | Author: Zhengru Ren
      | Date: May 20, 2016
      mask init:
      | invM_h = diag([1/m_h,1/m_h,1/m_h]);
  Lift wire : MarIn_blade/Lifting equipments (winch, wire, hook)/wire (changable length)  k=k_w1_s  c=d_w1_s
      settings: SourceProductName=MarIn (Blade)
  Sling {1..4} (4 alike) : MarIn_blade/Lifting equipments (winch, wire, hook)/wire (changable length)  k=k_w2_s  c=d_w2_s
      settings: SourceProductName=MarIn (Blade)
  Sum : Sum  Inputs=++++
  Sum1 : Sum  Inputs=++|
  Sum3 : Sum  Inputs=4
  Terminator1 : Terminator
  "position of connection point to the lift sling1{b}" : Constant  Value=posSling_s_b(:,1)
  "position of connection point to the lift sling1{b}1" : Constant  Value=posSling_s_b(:,4)
  "position of connection point to the lift sling2{b}" : Constant  Value=posSling_s_b(:,2)
  "position of connection point to the lift sling2{b}1" : Constant  Value=posSling_s_b(:,3)
  tau_sling : Outport
  wires:
  "nu(6DOF){bb}"/1 -> "External force(3DOF){n} nu{b} to Force&Torque(6DOF){b}"/4("nu{b}"), "External force(3DOF){n} nu{b} to Force&Torque(6DOF){b}1"/4("nu{b}"), "External force(3DOF){n} nu{b} to Force&Torque(6DOF){b}4"/4("nu{b}"), "External force(3DOF){n} nu{b} to Force&Torque(6DOF){b}5"/4("nu{b}")
  "position of connection point to the lift sling1{b}1"/1 -> "External force(3DOF){n} nu{b} to Force&Torque(6DOF){b}5"/1(pos_b)
  "External force(3DOF){n} nu{b} to Force&Torque(6DOF){b}"/1(tau_ex [6n X 1]) -> Sum3/4
  "eta(6DOF){n}"/1 -> "External force(3DOF){n} nu{b} to Force&Torque(6DOF){b}5"/3("eta{n}"), "External force(3DOF){n} nu{b} to Force&Torque(6DOF){b}"/3("eta{n}"), "External force(3DOF){n} nu{b} to Force&Torque(6DOF){b}1"/3("eta{n}"), "External force(3DOF){n} nu{b} to Force&Torque(6DOF){b}4"/3("eta{n}")
  "External force(3DOF){n} nu{b} to Force&Torque(6DOF){b}5"/1(tau_ex [6n X 1]) -> Sum3/1
  "position of connection point to the lift sling2{b}"/1 -> "External force(3DOF){n} nu{b} to Force&Torque(6DOF){b}"/1(pos_b)
  Sum3/1 -> tau_sling/1  "tau_sling"
  "External force(3DOF){n} nu{b} to Force&Torque(6DOF){b}4"/1(tau_ex [6n X 1]) -> Sum3/2
  [f_wire4_n] -> "External force(3DOF){n} nu{b} to Force&Torque(6DOF){b}5"/2("f_ex{n} [3 X n]")
  [f_wire3_n] -> "External force(3DOF){n} nu{b} to Force&Torque(6DOF){b}4"/2("f_ex{n} [3 X n]")
  "position of connection point to the lift sling2{b}1"/1 -> "External force(3DOF){n} nu{b} to Force&Torque(6DOF){b}4"/1(pos_b)
  "External force(3DOF){n} nu{b} to Force&Torque(6DOF){b}1"/3(nu_n[3 X 1]) -> [nuLiftwire1_n]
  "External force(3DOF){n} nu{b} to Force&Torque(6DOF){b}4"/2(pos_n[3 X 1]) -> [posLiftwire3_n]
  "position of connection point to the lift sling1{b}"/1 -> "External force(3DOF){n} nu{b} to Force&Torque(6DOF){b}1"/1(pos_b)
  "External force(3DOF){n} nu{b} to Force&Torque(6DOF){b}4"/3(nu_n[3 X 1]) -> [nuLiftwire3_n]
  [f_wire2_n] -> "External force(3DOF){n} nu{b} to Force&Torque(6DOF){b}"/2("f_ex{n} [3 X n]")
  "External force(3DOF){n} nu{b} to Force&Torque(6DOF){b}"/3(nu_n[3 X 1]) -> [nuLiftwire2_n]
  "External force(3DOF){n} nu{b} to Force&Torque(6DOF){b}"/2(pos_n[3 X 1]) -> [posLiftwire2_n]
  "External force(3DOF){n} nu{b} to Force&Torque(6DOF){b}1"/1(tau_ex [6n X 1]) -> Sum3/3
  "External force(3DOF){n} nu{b} to Force&Torque(6DOF){b}1"/2(pos_n[3 X 1]) -> [posLiftwire1_n]
  [f_wire1_n] -> "External force(3DOF){n} nu{b} to Force&Torque(6DOF){b}1"/2("f_ex{n} [3 X n]")
  Sling 4/2 -> [f_wire4_n]
  Sling 3/2 -> [f_wire3_n]
  Sling 4/1 -> Sum/4
  Sling 3/1 -> Sum/3
  [posLiftwire3_n] -> Sling 3/3
  [nuLiftwire3_n] -> Sling 3/4
  Hook/2(velHook) -> Sling 3/2, Sling 4/2, Sling 2/2, Sling 1/2, Lift wire/4
  Constant/1 -> Lift wire/5
  [posLiftwire1_n] -> Sling 1/3
  Sling 1/2 -> [f_wire1_n]
  [nuLiftwire1_n] -> Sling 1/4
  Sling 2/1 -> Sum/2
  Sling 2/2 -> [f_wire2_n]
  [posLiftwire2_n] -> Sling 2/3
  [nuLiftwire2_n] -> Sling 2/4
  Constant9/1 -> Sling 1/5, Sling 2/5, Sling 3/5, Sling 4/5
  Constant7/1 -> Lift wire/1
  Constant10/1 -> Lift wire/2
  Sum/1 -> Sum1/1
  Lift wire/2 -> Sum1/2
  Lift wire/1 -> Terminator1/1
  Sum1/1 -> Hook/1(total external force)
  Hook/1(posHook) -> Sling 3/1, Sling 4/1, Sling 2/1, Lift wire/3, Sling 1/1  "position of the hook"
  Constant4/1 -> Sling 2/6, Sling 1/6, Sling 3/6, Sling 4/6
  Constant6/1 -> Lift wire/6
  Sling 1/1 -> Sum/1
  [nuLiftwire4_n] -> Sling 4/4
  [posLiftwire4_n] -> Sling 4/3
  "External force(3DOF){n} nu{b} to Force&Torque(6DOF){b}5"/3(nu_n[3 X 1]) -> [nuLiftwire4_n]
  "External force(3DOF){n} nu{b} to Force&Torque(6DOF){b}5"/2(pos_n[3 X 1]) -> [posLiftwire4_n]

== system scale_model_model_control/Blade+Yoke1/thrusters ==
  "F_thrusters {b}" : Inport
  Demux : Demux
  Force(3DOF){b}2Force&Torque(6DOF){b}{,1..3} (4 alike) : MarIn_blade/Basic functions/Force(3DOF){b}2Force&Torque(6DOF){b}  posCOG_bb=posCOG_s
      settings: SourceProductName=MarIn (Blade)
  Sum3 : Sum  Inputs=4
  "position of connection point to thruster1{b}" : Constant  Value=posThruster_s_b(:,1)
  "position of connection point to thruster2{b}" : Constant  Value=posThruster_s_b(:,2)
  "position of connection point to thruster3{b}" : Constant  Value=posThruster_s_b(:,3)
  "position of connection point to thruster4{b}" : Constant  Value=posThruster_s_b(:,4)
  tau_thrusters : Outport
  wires:
  "position of connection point to thruster1{b}"/1 -> "Force(3DOF){b}2Force&Torque(6DOF){b}1"/1
  "position of connection point to thruster3{b}"/1 -> "Force(3DOF){b}2Force&Torque(6DOF){b}2"/1
  Sum3/1 -> tau_thrusters/1  "tau_thrusters"
  "position of connection point to thruster2{b}"/1 -> "Force(3DOF){b}2Force&Torque(6DOF){b}"/1
  "Force(3DOF){b}2Force&Torque(6DOF){b}"/1 -> Sum3/4
  "position of connection point to thruster4{b}"/1 -> "Force(3DOF){b}2Force&Torque(6DOF){b}3"/1
  "Force(3DOF){b}2Force&Torque(6DOF){b}3"/1 -> Sum3/1
  "Force(3DOF){b}2Force&Torque(6DOF){b}2"/1 -> Sum3/2
  "Force(3DOF){b}2Force&Torque(6DOF){b}1"/1 -> Sum3/3
  "F_thrusters {b}"/1 -> Demux/1
  Demux/4 -> "Force(3DOF){b}2Force&Torque(6DOF){b}3"/2
  Demux/3 -> "Force(3DOF){b}2Force&Torque(6DOF){b}2"/2
  Demux/1 -> "Force(3DOF){b}2Force&Torque(6DOF){b}1"/2
  Demux/2 -> "Force(3DOF){b}2Force&Torque(6DOF){b}"/2

== system scale_model_model_control/Blade+Yoke2/Signal Builder2 ==
  Demux : Demux  Tag=STV Demux  Outputs=1
      settings: DisplayOption=none
  FromWs : FromWorkspace  Tag=STV FromWs  VariableName=tuvar
      SigBuilderData=|
      | common.afterFinalStr = 'Extrapolate'
      | common.sampleTime = 0
      | dataSet.timeRange = [0 10]
      | dataSet.name = 'Group 1'
      | sbobj.Groups.Name = 'Group 1'
      | sbobj.Groups.Signals.Name = 'Signal 1'
      | sbobj.Groups.Signals.XData = [0 2 2 2.1 2.1 10]
      | sbobj.Groups.Signals.YData = [0 0 1 1 0 0]
  Signal 1 : Outport  Tag=STV Outport
  wires:
  Demux/1 -> Signal 1/1
  FromWs/1 -> Demux/1

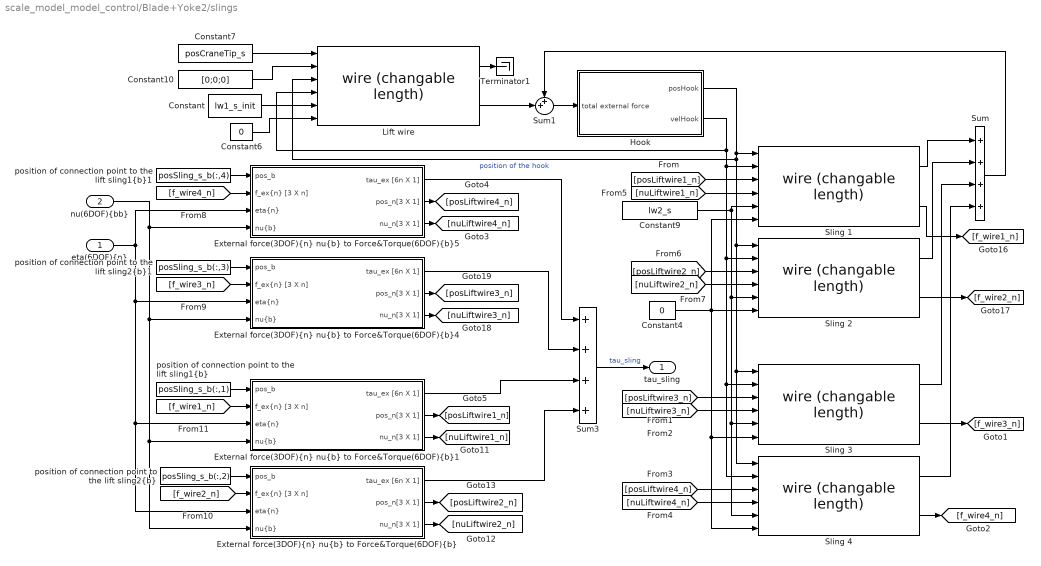
== system scale_model_model_control/Blade+Yoke2/slings ==
  "eta(6DOF){n}" : Inport
  "nu(6DOF){bb}" : Inport  Port=2
  Constant : Constant  Value=lw1_s_init
  Constant10 : Constant  Value=[0;0;0]
  Constant4 : Constant  Value=0
  Constant6 : Constant  Value=0
  Constant7 : Constant  Value=posCraneTip_s
  Constant9 : Constant  Value=lw2_s
  "External force(3DOF){n} nu{b} to Force&Torque(6DOF){b}" : Subsystem  AncestorBlock=MarIn_blade/Basic functions/External force(3DOF){n} nu{b} to Force&Torque(6DOF){b}  mask(External force(3DOF){n} nu{b} to Force&Torque(6DOF){b}){}
      mask help:
      | Translate position and velocity in {b} to {n}.
      |
      |
      | Author: Zhengru Ren
      | Date: April 22, 2017
  "External force(3DOF){n} nu{b} to Force&Torque(6DOF){b}1" : Subsystem  AncestorBlock=MarIn_blade/Basic functions/External force(3DOF){n} nu{b} to Force&Torque(6DOF){b}  mask(External force(3DOF){n} nu{b} to Force&Torque(6DOF){b}){}
      mask help:
      | Translate position and velocity in {b} to {n}.
      |
      |
      | Author: Zhengru Ren
      | Date: April 22, 2017
  "External force(3DOF){n} nu{b} to Force&Torque(6DOF){b}4" : Subsystem  AncestorBlock=MarIn_blade/Basic functions/External force(3DOF){n} nu{b} to Force&Torque(6DOF){b}  mask(External force(3DOF){n} nu{b} to Force&Torque(6DOF){b}){}
      mask help:
      | Translate position and velocity in {b} to {n}.
      |
      |
      | Author: Zhengru Ren
      | Date: April 22, 2017
  "External force(3DOF){n} nu{b} to Force&Torque(6DOF){b}5" : Subsystem  AncestorBlock=MarIn_blade/Basic functions/External force(3DOF){n} nu{b} to Force&Torque(6DOF){b}  mask(External force(3DOF){n} nu{b} to Force&Torque(6DOF){b}){}
      mask help:
      | Translate position and velocity in {b} to {n}.
      |
      |
      | Author: Zhengru Ren
      | Date: April 22, 2017
  Hook : Subsystem  AncestorBlock=|  mask(Hook){m_h=m_h_s, p_h_init=p_h_s_init, p_h_dot_init=p_h_dot_s_init}
      | MarIn_blade/Lifting equipments
      | (winch, wire, hook)/Hook
      mask prompts: m_h "Hook mass (m_h) [kg]"; p_h_init "Initial position of the hook"; p_h_dot_init "Initial velocity of the hook"
      mask help:
      | Used to simulate a hook.
      |
      | Author: Zhengru Ren
      | Date: May 20, 2016
      mask init:
      | invM_h = diag([1/m_h,1/m_h,1/m_h]);
  Lift wire : MarIn_blade/Lifting equipments (winch, wire, hook)/wire (changable length)  k=k_w1_s  c=d_w1_s
      settings: SourceProductName=MarIn (Blade)
  Sling {1..4} (4 alike) : MarIn_blade/Lifting equipments (winch, wire, hook)/wire (changable length)  k=k_w2_s  c=d_w2_s
      settings: SourceProductName=MarIn (Blade)
  Sum : Sum  Inputs=++++
  Sum1 : Sum  Inputs=++|
  Sum3 : Sum  Inputs=4
  Terminator1 : Terminator
  "position of connection point to the lift sling1{b}" : Constant  Value=posSling_s_b(:,1)
  "position of connection point to the lift sling1{b}1" : Constant  Value=posSling_s_b(:,4)
  "position of connection point to the lift sling2{b}" : Constant  Value=posSling_s_b(:,2)
  "position of connection point to the lift sling2{b}1" : Constant  Value=posSling_s_b(:,3)
  tau_sling : Outport
  wires:
  "nu(6DOF){bb}"/1 -> "External force(3DOF){n} nu{b} to Force&Torque(6DOF){b}"/4("nu{b}"), "External force(3DOF){n} nu{b} to Force&Torque(6DOF){b}1"/4("nu{b}"), "External force(3DOF){n} nu{b} to Force&Torque(6DOF){b}4"/4("nu{b}"), "External force(3DOF){n} nu{b} to Force&Torque(6DOF){b}5"/4("nu{b}")
  "position of connection point to the lift sling1{b}1"/1 -> "External force(3DOF){n} nu{b} to Force&Torque(6DOF){b}5"/1(pos_b)
  "External force(3DOF){n} nu{b} to Force&Torque(6DOF){b}"/1(tau_ex [6n X 1]) -> Sum3/4
  "eta(6DOF){n}"/1 -> "External force(3DOF){n} nu{b} to Force&Torque(6DOF){b}5"/3("eta{n}"), "External force(3DOF){n} nu{b} to Force&Torque(6DOF){b}"/3("eta{n}"), "External force(3DOF){n} nu{b} to Force&Torque(6DOF){b}1"/3("eta{n}"), "External force(3DOF){n} nu{b} to Force&Torque(6DOF){b}4"/3("eta{n}")
  "External force(3DOF){n} nu{b} to Force&Torque(6DOF){b}5"/1(tau_ex [6n X 1]) -> Sum3/1
  "position of connection point to the lift sling2{b}"/1 -> "External force(3DOF){n} nu{b} to Force&Torque(6DOF){b}"/1(pos_b)
  Sum3/1 -> tau_sling/1  "tau_sling"
  "External force(3DOF){n} nu{b} to Force&Torque(6DOF){b}4"/1(tau_ex [6n X 1]) -> Sum3/2
  [f_wire4_n] -> "External force(3DOF){n} nu{b} to Force&Torque(6DOF){b}5"/2("f_ex{n} [3 X n]")
  [f_wire3_n] -> "External force(3DOF){n} nu{b} to Force&Torque(6DOF){b}4"/2("f_ex{n} [3 X n]")
  "position of connection point to the lift sling2{b}1"/1 -> "External force(3DOF){n} nu{b} to Force&Torque(6DOF){b}4"/1(pos_b)
  "External force(3DOF){n} nu{b} to Force&Torque(6DOF){b}1"/3(nu_n[3 X 1]) -> [nuLiftwire1_n]
  "External force(3DOF){n} nu{b} to Force&Torque(6DOF){b}4"/2(pos_n[3 X 1]) -> [posLiftwire3_n]
  "position of connection point to the lift sling1{b}"/1 -> "External force(3DOF){n} nu{b} to Force&Torque(6DOF){b}1"/1(pos_b)
  "External force(3DOF){n} nu{b} to Force&Torque(6DOF){b}4"/3(nu_n[3 X 1]) -> [nuLiftwire3_n]
  [f_wire2_n] -> "External force(3DOF){n} nu{b} to Force&Torque(6DOF){b}"/2("f_ex{n} [3 X n]")
  "External force(3DOF){n} nu{b} to Force&Torque(6DOF){b}"/3(nu_n[3 X 1]) -> [nuLiftwire2_n]
  "External force(3DOF){n} nu{b} to Force&Torque(6DOF){b}"/2(pos_n[3 X 1]) -> [posLiftwire2_n]
  "External force(3DOF){n} nu{b} to Force&Torque(6DOF){b}1"/1(tau_ex [6n X 1]) -> Sum3/3
  "External force(3DOF){n} nu{b} to Force&Torque(6DOF){b}1"/2(pos_n[3 X 1]) -> [posLiftwire1_n]
  [f_wire1_n] -> "External force(3DOF){n} nu{b} to Force&Torque(6DOF){b}1"/2("f_ex{n} [3 X n]")
  Sling 4/2 -> [f_wire4_n]
  Sling 3/2 -> [f_wire3_n]
  Sling 4/1 -> Sum/4
  Sling 3/1 -> Sum/3
  [posLiftwire3_n] -> Sling 3/3
  [nuLiftwire3_n] -> Sling 3/4
  Hook/2(velHook) -> Sling 3/2, Sling 4/2, Sling 2/2, Sling 1/2, Lift wire/4
  Constant/1 -> Lift wire/5
  [posLiftwire1_n] -> Sling 1/3
  Sling 1/2 -> [f_wire1_n]
  [nuLiftwire1_n] -> Sling 1/4
  Sling 2/1 -> Sum/2
  Sling 2/2 -> [f_wire2_n]
  [posLiftwire2_n] -> Sling 2/3
  [nuLiftwire2_n] -> Sling 2/4
  Constant9/1 -> Sling 1/5, Sling 2/5, Sling 3/5, Sling 4/5
  Constant7/1 -> Lift wire/1
  Constant10/1 -> Lift wire/2
  Sum/1 -> Sum1/1
  Lift wire/2 -> Sum1/2
  Lift wire/1 -> Terminator1/1
  Sum1/1 -> Hook/1(total external force)
  Hook/1(posHook) -> Sling 3/1, Sling 4/1, Sling 2/1, Lift wire/3, Sling 1/1  "position of the hook"
  Constant4/1 -> Sling 2/6, Sling 1/6, Sling 3/6, Sling 4/6
  Constant6/1 -> Lift wire/6
  Sling 1/1 -> Sum/1
  [nuLiftwire4_n] -> Sling 4/4
  [posLiftwire4_n] -> Sling 4/3
  "External force(3DOF){n} nu{b} to Force&Torque(6DOF){b}5"/3(nu_n[3 X 1]) -> [nuLiftwire4_n]
  "External force(3DOF){n} nu{b} to Force&Torque(6DOF){b}5"/2(pos_n[3 X 1]) -> [posLiftwire4_n]

== system scale_model_model_control/Blade+Yoke2/thrusters ==
  "F_thrusters {b}" : Inport
  Demux : Demux
  Force(3DOF){b}2Force&Torque(6DOF){b}{,1..3} (4 alike) : MarIn_blade/Basic functions/Force(3DOF){b}2Force&Torque(6DOF){b}  posCOG_bb=posCOG_s
      settings: SourceProductName=MarIn (Blade)
  Sum3 : Sum  Inputs=4
  "position of connection point to thruster1{b}" : Constant  Value=posThruster_s_b(:,1)
  "position of connection point to thruster2{b}" : Constant  Value=posThruster_s_b(:,2)
  "position of connection point to thruster3{b}" : Constant  Value=posThruster_s_b(:,3)
  "position of connection point to thruster4{b}" : Constant  Value=posThruster_s_b(:,4)
  tau_thrusters : Outport
  wires:
  "position of connection point to thruster1{b}"/1 -> "Force(3DOF){b}2Force&Torque(6DOF){b}1"/1
  "position of connection point to thruster3{b}"/1 -> "Force(3DOF){b}2Force&Torque(6DOF){b}2"/1
  Sum3/1 -> tau_thrusters/1  "tau_thrusters"
  "position of connection point to thruster2{b}"/1 -> "Force(3DOF){b}2Force&Torque(6DOF){b}"/1
  "Force(3DOF){b}2Force&Torque(6DOF){b}"/1 -> Sum3/4
  "position of connection point to thruster4{b}"/1 -> "Force(3DOF){b}2Force&Torque(6DOF){b}3"/1
  "Force(3DOF){b}2Force&Torque(6DOF){b}3"/1 -> Sum3/1
  "Force(3DOF){b}2Force&Torque(6DOF){b}2"/1 -> Sum3/2
  "Force(3DOF){b}2Force&Torque(6DOF){b}1"/1 -> Sum3/3
  "F_thrusters {b}"/1 -> Demux/1
  Demux/4 -> "Force(3DOF){b}2Force&Torque(6DOF){b}3"/2
  Demux/3 -> "Force(3DOF){b}2Force&Torque(6DOF){b}2"/2
  Demux/1 -> "Force(3DOF){b}2Force&Torque(6DOF){b}1"/2
  Demux/2 -> "Force(3DOF){b}2Force&Torque(6DOF){b}"/2

== system scale_model_model_control/Blade+Yoke3/Signal Builder2 ==
  Demux : Demux  Tag=STV Demux  Outputs=1
      settings: DisplayOption=none
  FromWs : FromWorkspace  Tag=STV FromWs  VariableName=tuvar
      SigBuilderData=|
      | common.afterFinalStr = 'Extrapolate'
      | common.sampleTime = 0
      | dataSet.timeRange = [0 10]
      | dataSet.name = 'Group 1'
      | sbobj.Groups.Name = 'Group 1'
      | sbobj.Groups.Signals.Name = 'Signal 1'
      | sbobj.Groups.Signals.XData = [0 2 2 2.1 2.1 10]
      | sbobj.Groups.Signals.YData = [0 0 1 1 0 0]
  Signal 1 : Outport  Tag=STV Outport
  wires:
  Demux/1 -> Signal 1/1
  FromWs/1 -> Demux/1
